simulink model "sb_control"  (R2014a)
settings: Solver=FixedStepDiscrete  StartTime=0.0  StopTime=3  FixedStep=Ts  MaxStep=1/60  RelTol=1e-4
PreLoadFcn:
  | load('synchbreaker_data');
StartFcn:
  | tic;
StopFcn:
  | toc;
values from neighbouring files (symbols this model uses):
  d1 = 0.04    [synchbreaker_data.mat]
  Ts = 4e-05    [synchbreaker_data.mat]
libraries: simulink x2
settings Model: RequirementInfo={'other' 'D:\CVS_Sandbox\P-MLSPG-20171\JIN002 - LPD Modelling\LPD Models\T1702v4_REQM_LINK.doc' '@Simulink_requirement_item_1' 'true' 'Update WR21 automatic synchronisation breaker for use on the LPD model.' '' } %GIDa_3ffb9889_e7fc_4053_bde8_e524ad01eccd  Creator=gdudgeon  LastModifiedBy=cosorio
settings DataIOCC: SaveOutput=off  SaveTime=off
settings OptimizationCC: ExpressionDepthLimit=2147483647
settings DebuggingCC: UnderspecifiedInitializationDetection=Classic  FcnCallInpInsideContextMsg=UseLocalSettings  StateNameClashWarn=warning
settings SFSimCC: SimParseCustomCode=off
settings GRTTargetCC: CombineOutputUpdateFcns=off  GRTInterface=on

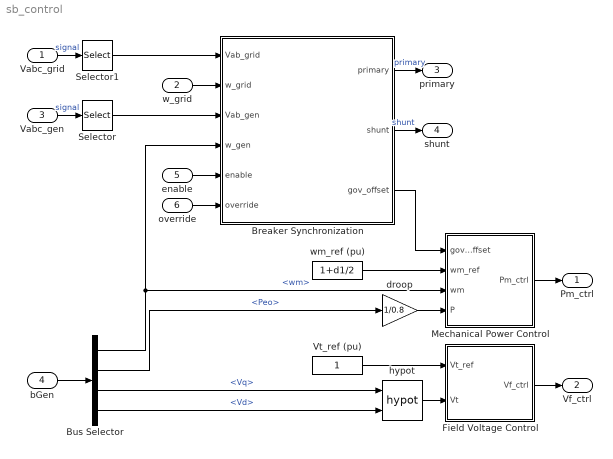
== system sb_control ==
  Vabc_grid : Inport  OutDataTypeStr=double  PortDimensions=3  SampleTime=Ts
  w_grid : Inport  Port=2  OutDataTypeStr=double  PortDimensions=1  SampleTime=Ts
  Vabc_gen : Inport  Port=3  OutDataTypeStr=double  PortDimensions=3  SampleTime=Ts
  bGen : Inport  Port=4  OutDataTypeStr=Bus: GenDataBus  SampleTime=[4.0000000000000003e-05,0]
  enable : Inport  Port=5  OutDataTypeStr=double  PortDimensions=1  SampleTime=Ts
  override : Inport  Port=6  OutDataTypeStr=double  PortDimensions=1  SampleTime=Ts
  Breaker Synchronization : Stateflow chart  TreatAsAtomicUnit=on
  Bus Selector : BusSelector  OutputSignals=wm,Peo,Vq,Vd
  Field Voltage Control : Subsystem
  Mechanical Power Control : Subsystem
  Selector : Selector  InputPortWidth=3  Indices=[1]
  Selector1 : Selector  InputPortWidth=3  Indices=[1]
  Vt_ref (pu) : Constant  SampleTime=Ts
  droop : Gain  Gain=1/0.8
  hypot : Math  Operator=hypot  SaturateOnIntegerOverflow=on
  wm_ref (pu) : Constant  Value=1+d1/2  SampleTime=Ts
  Pm_ctrl : Outport  OutDataTypeStr=double  PortDimensions=1  SampleTime=Ts
  Vf_ctrl : Outport  Port=2  OutDataTypeStr=double  PortDimensions=1  SampleTime=Ts
  primary : Outport  Port=3  OutDataTypeStr=double  PortDimensions=1  SampleTime=Ts
  shunt : Outport  Port=4  OutDataTypeStr=double  PortDimensions=1  SampleTime=Ts
  wires:
  override/1 -> Breaker Synchronization/6(override)
  Breaker Synchronization/3(gov_offset) -> Mechanical Power Control/1(gov_offset)
  Breaker Synchronization/1(primary) -> primary/1  "primary"
  enable/1 -> Breaker Synchronization/5(enable)
  Vabc_gen/1 -> Selector/1  "signal"
  Selector/1 -> Breaker Synchronization/3(Vab_gen)
  Vabc_grid/1 -> Selector1/1  "signal"
  Selector1/1 -> Breaker Synchronization/1(Vab_grid)
  Bus Selector/1 -> Breaker Synchronization/4(w_gen), Mechanical Power Control/3(wm)  "<wm>"
  wm_ref (pu)/1 -> Mechanical Power Control/2(wm_ref)
  Mechanical Power Control/1(Pm_ctrl) -> Pm_ctrl/1
  Vt_ref (pu)/1 -> Field Voltage Control/1(Vt_ref)
  Field Voltage Control/1(Vf_ctrl) -> Vf_ctrl/1
  droop/1 -> Mechanical Power Control/4(P)
  bGen/1 -> Bus Selector/1
  hypot/1 -> Field Voltage Control/2(Vt)
  w_grid/1 -> Breaker Synchronization/2(w_grid)
  Bus Selector/2 -> droop/1  "<Peo>"
  Bus Selector/3 -> hypot/1  "<Vq>"
  Bus Selector/4 -> hypot/2  "<Vd>"
  Breaker Synchronization/2(shunt) -> shunt/1  "shunt"

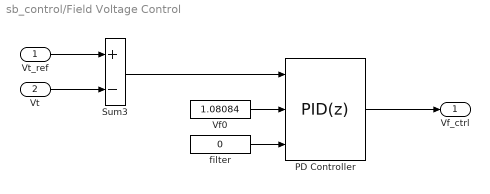
== system sb_control/Field Voltage Control ==
  Vt_ref : Inport
  Vt : Inport  Port=2
  PD Controller : simulink/Continuous/PID Controller  Controller=PID  TimeDomain=Discrete-time  SampleTime=Ts  IntegratorMethod=Forward Euler  FilterMethod=Forward Euler  Form=Parallel  P=200  I=250  D=-1.8  N=100  InitialConditionSource=external  InitialConditionForIntegrator=0  InitialConditionForFilter=0  ExternalReset=none  LimitOutput=off  UpperSaturationLimit=inf  LowerSaturationLimit=-inf  LinearizeAsGain=on  AntiWindupMode=none  Kb=1  TrackingMode=off  Kt=1  PParamMin=[]  PParamMax=[]  IParamMin=[]  IParamMax=[]  DParamMin=[]  DParamMax=[]  NParamMin=[]  NParamMax=[]  KbParamMin=[]  KbParamMax=[]  KtParamMin=[]  KtParamMax=[]  POutMin=[]  POutMax=[]  IOutMin=[]  IOutMax=[]  DOutMin=[]  DOutMax=[]  NOutMin=[]  NOutMax=[]  KbOutMin=[]  KbOutMax=[]  KtOutMin=[]  KtOutMax=[]  IntegratorOutMin=[]  IntegratorOutMax=[]  FilterOutMin=[]  FilterOutMax=[]  SumOutMin=[]  SumOutMax=[]  SumI1OutMin=[]  SumI1OutMax=[]  SumI2OutMin=[]  SumI2OutMax=[]  SumI3OutMin=[]  SumI3OutMax=[]  SumDOutMin=[]  SumDOutMax=[]  SaturationOutMin=[]  SaturationOutMax=[]  IntegratorContinuousStateAttributes=''  IntegratorStateMustResolveToSignalObject=off  IntegratorRTWStateStorageClass=Auto  FilterContinuousStateAttributes=''  FilterStateMustResolveToSignalObject=off  FilterRTWStateStorageClass=Auto
  Sum3 : Sum  Inputs=+-
  Vf0 : Constant  Value=1.08084  SampleTime=Ts
  filter : Constant  Value=0  SampleTime=Ts
  Vf_ctrl : Outport
  wires:
  filter/1 -> PD Controller/3
  PD Controller/1 -> Vf_ctrl/1
  Vf0/1 -> PD Controller/2
  Vt/1 -> Sum3/2
  Vt_ref/1 -> Sum3/1
  Sum3/1 -> PD Controller/1

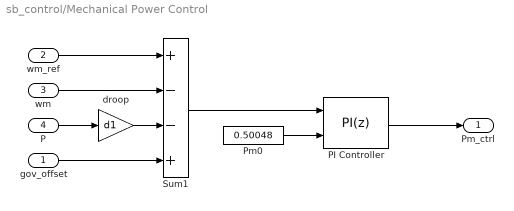
== system sb_control/Mechanical Power Control ==
  gov_offset : Inport
  wm_ref : Inport  Port=2
  wm : Inport  Port=3
  P : Inport  Port=4
  PI Controller : simulink/Continuous/PID Controller  Controller=PI  TimeDomain=Discrete-time  SampleTime=Ts  IntegratorMethod=Forward Euler  FilterMethod=Forward Euler  Form=Parallel  P=400  I=200  D=0.000000000000000  N=99.900066633346043  InitialConditionSource=external  InitialConditionForIntegrator=0  InitialConditionForFilter=0  ExternalReset=none  LimitOutput=off  UpperSaturationLimit=inf  LowerSaturationLimit=-inf  LinearizeAsGain=on  AntiWindupMode=none  Kb=1  TrackingMode=off  Kt=1  PParamMin=[]  PParamMax=[]  IParamMin=[]  IParamMax=[]  DParamMin=[]  DParamMax=[]  NParamMin=[]  NParamMax=[]  KbParamMin=[]  KbParamMax=[]  KtParamMin=[]  KtParamMax=[]  POutMin=[]  POutMax=[]  IOutMin=[]  IOutMax=[]  DOutMin=[]  DOutMax=[]  NOutMin=[]  NOutMax=[]  KbOutMin=[]  KbOutMax=[]  KtOutMin=[]  KtOutMax=[]  IntegratorOutMin=[]  IntegratorOutMax=[]  FilterOutMin=[]  FilterOutMax=[]  SumOutMin=[]  SumOutMax=[]  SumI1OutMin=[]  SumI1OutMax=[]  SumI2OutMin=[]  SumI2OutMax=[]  SumI3OutMin=[]  SumI3OutMax=[]  SumDOutMin=[]  SumDOutMax=[]  SaturationOutMin=[]  SaturationOutMax=[]  IntegratorContinuousStateAttributes=''  IntegratorStateMustResolveToSignalObject=off  IntegratorRTWStateStorageClass=Auto  FilterContinuousStateAttributes=''  FilterStateMustResolveToSignalObject=off  FilterRTWStateStorageClass=Auto
  Pm0 : Constant  Value=0.50048  SampleTime=Ts
  Sum1 : Sum  Inputs=+--+
  droop : Gain  Gain=d1
  Pm_ctrl : Outport
  wires:
  Pm0/1 -> PI Controller/2
  PI Controller/1 -> Pm_ctrl/1
  wm/1 -> Sum1/2
  droop/1 -> Sum1/3
  gov_offset/1 -> Sum1/4
  wm_ref/1 -> Sum1/1
  Sum1/1 -> PI Controller/1
  P/1 -> droop/1

== stateflow chart sb_control/Breaker Synchronization ==
  settings: updateMethod=DISCRETE  sampleTime=Ts
  state Synchronize
    state PhaseSynch [parallel]
      settings: executionOrder=1
      state InitPhaseSynch
        entry:
        ready = 0;
        primary = 0;
        shunt = 1;
      state Wait
      state PhaseSynchCheck1
        du: Vab_e = Vab_gen - Vab_grid;
      state Connect
        entry:
        ready = 1;
        primary = 1;
        shunt = 0;
      state PhaseSynchCheck2
        du: Vab_e = Vab_gen - Vab_grid;
      (default) -> InitPhaseSynch
      InitPhaseSynch -> Wait : [abs(w_e) < w_tol]
      Wait -> PhaseSynchCheck1 [order 1] : [after(ceil(0.5/Ts),tick)]
      PhaseSynchCheck1 -> Wait [order 1] : [abs(w_e) >= w_tol]
      Wait -> InitPhaseSynch [order 2] : [abs(w_e) >= w_tol]
      PhaseSynchCheck2 -> PhaseSynchCheck1 [order 1] : [abs(Vab_e) >= v_tol]
      PhaseSynchCheck1 -> PhaseSynchCheck2 [order 2] : [abs(Vab_e) < v_tol]
      PhaseSynchCheck2 -> Connect [order 2] : [after(ceil((0.24/60)/Ts),tick) ]
    state FrequencySynch [parallel]
      settings: executionOrder=2
      state InitReadyConnect
        entry:
        gov_offset = 0;
        w_e = 1;
      state SetFrequencyOffset
        during:
        w_e = (w_grid + w_offset) - w_gen;
        y = y_prev+Ts*w_e;
        gov_offset = ki*y + kp*w_e;
        y_prev = y;
      SetFrequencyOffset -> InitReadyConnect : [ready]
      InitReadyConnect -> SetFrequencyOffset : [!ready]
      (default) -> InitReadyConnect
  state Connected
    entry:
    primary = 1;
    shunt = 0;
    gov_offset = 0;
  state Disconnected
    entry:
    primary = 0;
    shunt = 1;
    gov_offset = 0;
  Synchronize -> Connected [order 1] : [override]
  Disconnected -> Synchronize [order 2] : [enable]
  Synchronize -> Disconnected [order 2] : [!enable]
  Connected -> Disconnected : [!override]
  (default) -> Connected
  Disconnected -> Connected [order 1] : [override]
  data: primary output double size=1 =1; shunt output double size=1 =1; Vab_grid input double size=1; w_grid input double size=1; Vab_gen input double size=1; w_gen input double size=1; gov_offset output double =0; Vab_e local double; w_e local double =1; ready local double =0; y local double =0; y_prev local double =0; enable input double size=1; w_offset local double =0.005; ki local double =50; v_tol local double =0.005; w_tol local double =0.005; kp local double =10; override input double size=1; Ts parameter double size=1 =Ts
